simulink model "Spring"  (R2018b)
settings: Solver=FixedStepAuto  StartTime=0.0  StopTime=20  FixedStep=0.1  RelTol=1e-3
undefined symbols (not defined in the file): c, k1, k2, m, x0
settings Model: Creator=ilab  LastModifiedBy=ilab

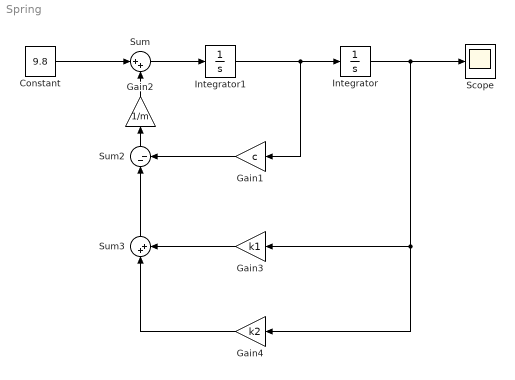
== system Spring ==
  Constant : Constant  Value=9.8
  Gain1 : Gain  Gain=c
  Gain2 : Gain  Gain=1/m
  Gain3 : Gain  Gain=k1
  Gain4 : Gain  Gain=k2
  Integrator : Integrator  InitialCondition=x0
  Integrator1 : Integrator
  Scope : Scope
  Sum : Sum  Inputs=|++
  Sum2 : Sum  Inputs=|--
  Sum3 : Sum  Inputs=|++
  wires:
  Sum/1 -> Integrator1/1
  Integrator1/1 -> Gain1/1, Integrator/1
  Constant/1 -> Sum/1
  Integrator/1 -> Gain3/1, Gain4/1, Scope/1
  Sum2/1 -> Gain2/1
  Gain1/1 -> Sum2/2
  Sum3/1 -> Sum2/1
  Gain3/1 -> Sum3/2
  Gain4/1 -> Sum3/1
  Gain2/1 -> Sum/2
